simulink model "TST_PTOSwt_DD"  (R2016b)
settings: Solver=FixedStepDiscrete  StartTime=0.0  StopTime=0.1  FixedStep=sampleTime  RelTol=1e-3
values from neighbouring files (symbols this model uses):
  testCase = 1    [initTST_PTOSwt_DD_001.m]
libraries: simulink x2
settings Model: Creator=guofang02  LastModifiedBy=guofang02
settings DebuggingCC: SignalRangeChecking=error

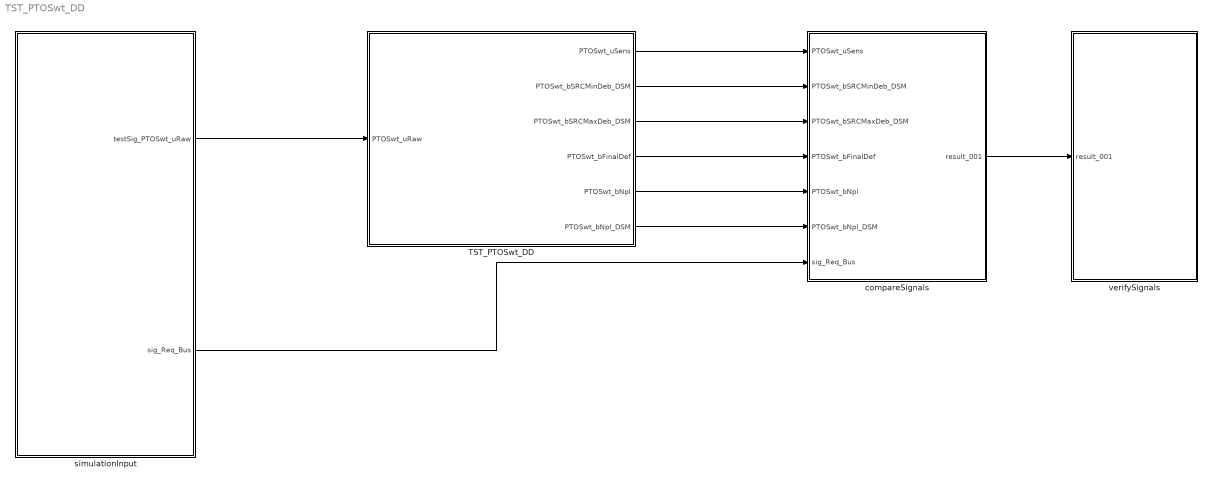
== system TST_PTOSwt_DD ==
  TST_PTOSwt_DD : Subsystem
  compareSignals : Subsystem
  simulationInput : Subsystem
  verifySignals : Subsystem
  wires:
  simulationInput/1(testSig_PTOSwt_uRaw) -> TST_PTOSwt_DD/1(PTOSwt_uRaw)
  TST_PTOSwt_DD/1(PTOSwt_uSens) -> compareSignals/1(PTOSwt_uSens)
  TST_PTOSwt_DD/2(PTOSwt_bSRCMinDeb_DSM) -> compareSignals/2(PTOSwt_bSRCMinDeb_DSM)
  TST_PTOSwt_DD/3(PTOSwt_bSRCMaxDeb_DSM) -> compareSignals/3(PTOSwt_bSRCMaxDeb_DSM)
  TST_PTOSwt_DD/4(PTOSwt_bFinalDef) -> compareSignals/4(PTOSwt_bFinalDef)
  TST_PTOSwt_DD/5(PTOSwt_bNpl) -> compareSignals/5(PTOSwt_bNpl)
  TST_PTOSwt_DD/6(PTOSwt_bNpl_DSM) -> compareSignals/6(PTOSwt_bNpl_DSM)
  simulationInput/2(sig_Req_Bus) -> compareSignals/7(sig_Req_Bus)
  compareSignals/1(result_001) -> verifySignals/1(result_001)

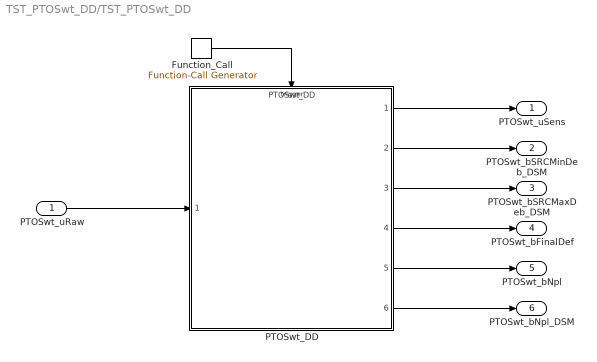
== system TST_PTOSwt_DD/TST_PTOSwt_DD ==
  PTOSwt_uRaw : Inport
  Function_Call : simulink/Ports & Subsystems/Function-Call Generator  sample_time=sampleTime  numberOfIterations=1
  PTOSwt_DD : ModelReference  ModelNameDialog=PTOSwt_DD  ModelReferenceVersion=1.16  TriggerPortName=function  TriggerPortTriggerType=function-call  TriggerPortStatesWhenEnabling=held
  PTOSwt_uSens : Outport
  PTOSwt_bSRCMinDeb_DSM : Outport  Port=2
  PTOSwt_bSRCMaxDeb_DSM : Outport  Port=3
  PTOSwt_bFinalDef : Outport  Port=4
  PTOSwt_bNpl : Outport  Port=5
  PTOSwt_bNpl_DSM : Outport  Port=6
  wires:
  Function_Call/1 -> PTOSwt_DD/Trigger
  PTOSwt_uRaw/1 -> PTOSwt_DD/1
  PTOSwt_DD/1 -> PTOSwt_uSens/1
  PTOSwt_DD/2 -> PTOSwt_bSRCMinDeb_DSM/1
  PTOSwt_DD/3 -> PTOSwt_bSRCMaxDeb_DSM/1
  PTOSwt_DD/4 -> PTOSwt_bFinalDef/1
  PTOSwt_DD/5 -> PTOSwt_bNpl/1
  PTOSwt_DD/6 -> PTOSwt_bNpl_DSM/1

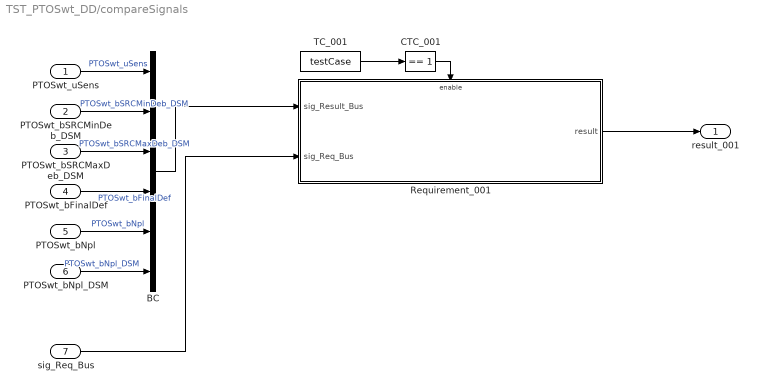
== system TST_PTOSwt_DD/compareSignals ==
  PTOSwt_uSens : Inport
  PTOSwt_bSRCMinDeb_DSM : Inport  Port=2
  PTOSwt_bSRCMaxDeb_DSM : Inport  Port=3
  PTOSwt_bFinalDef : Inport  Port=4
  PTOSwt_bNpl : Inport  Port=5
  PTOSwt_bNpl_DSM : Inport  Port=6
  sig_Req_Bus : Inport  Port=7
  BC : BusCreator  Inputs=6
  CTC_001 : simulink/Logic and Bit Operations/Compare To Constant  relop===  const=1  OutDataTypeStr=boolean
  Requirement_001 : Subsystem
  TC_001 : Constant  Value=testCase
  result_001 : Outport
  wires:
  PTOSwt_uSens/1 -> BC/1  "PTOSwt_uSens"
  PTOSwt_bSRCMinDeb_DSM/1 -> BC/2  "PTOSwt_bSRCMinDeb_DSM"
  PTOSwt_bSRCMaxDeb_DSM/1 -> BC/3  "PTOSwt_bSRCMaxDeb_DSM"
  PTOSwt_bFinalDef/1 -> BC/4  "PTOSwt_bFinalDef"
  PTOSwt_bNpl/1 -> BC/5  "PTOSwt_bNpl"
  PTOSwt_bNpl_DSM/1 -> BC/6  "PTOSwt_bNpl_DSM"
  TC_001/1 -> CTC_001/1
  CTC_001/1 -> Requirement_001/Enable
  sig_Req_Bus/1 -> Requirement_001/2(sig_Req_Bus)
  BC/1 -> Requirement_001/1(sig_Result_Bus)
  Requirement_001/1(result) -> result_001/1

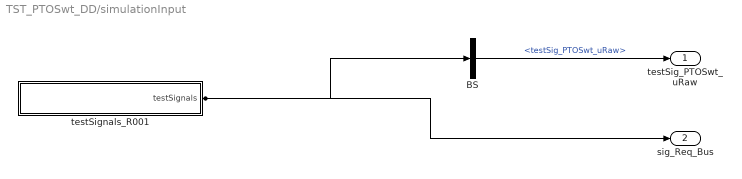
== system TST_PTOSwt_DD/simulationInput ==
  BS : BusSelector  OutputSignals=testSig_PTOSwt_uRaw
  testSignals_R001 : Subsystem
  testSig_PTOSwt_uRaw : Outport
  sig_Req_Bus : Outport  Port=2
  wires:
  BS/1 -> testSig_PTOSwt_uRaw/1  "<testSig_PTOSwt_uRaw>"
  testSignals_R001/1(testSignals) -> BS/1, sig_Req_Bus/1

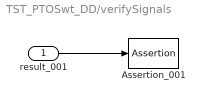
== system TST_PTOSwt_DD/verifySignals ==
  result_001 : Inport
  Assertion_001 : Assertion
  wires:
  result_001/1 -> Assertion_001/1

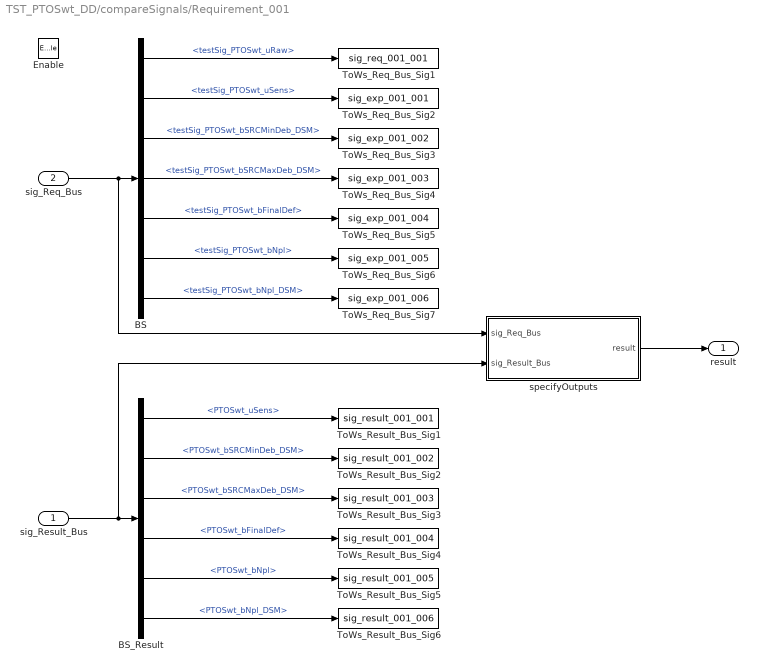
== system TST_PTOSwt_DD/compareSignals/Requirement_001 ==
  sig_Result_Bus : Inport
  sig_Req_Bus : Inport  Port=2
  Enable : EnablePort
  BS : BusSelector  OutputSignals=testSig_PTOSwt_uRaw,testSig_PTOSwt_uSens,testSig_PTOSwt_bSRCMinDeb_DSM,testSig_PTOSwt_bSRCMaxDeb_DSM,testSig_PTOSwt_bFinalDef,testSig_PTOSwt_bNpl,testSig_PTOSwt_bNpl_DSM
  BS_Result : BusSelector  OutputSignals=PTOSwt_uSens,PTOSwt_bSRCMinDeb_DSM,PTOSwt_bSRCMaxDeb_DSM,PTOSwt_bFinalDef,PTOSwt_bNpl,PTOSwt_bNpl_DSM
  ToWs_Req_Bus_Sig1 : ToWorkspace  VariableName=sig_req_001_001  SaveFormat=Structure With Time
  ToWs_Req_Bus_Sig2 : ToWorkspace  VariableName=sig_exp_001_001  SaveFormat=Structure With Time
  ToWs_Req_Bus_Sig3 : ToWorkspace  VariableName=sig_exp_001_002  SaveFormat=Structure With Time
  ToWs_Req_Bus_Sig4 : ToWorkspace  VariableName=sig_exp_001_003  SaveFormat=Structure With Time
  ToWs_Req_Bus_Sig5 : ToWorkspace  VariableName=sig_exp_001_004  SaveFormat=Structure With Time
  ToWs_Req_Bus_Sig6 : ToWorkspace  VariableName=sig_exp_001_005  SaveFormat=Structure With Time
  ToWs_Req_Bus_Sig7 : ToWorkspace  VariableName=sig_exp_001_006  SaveFormat=Structure With Time
  ToWs_Result_Bus_Sig1 : ToWorkspace  VariableName=sig_result_001_001  SaveFormat=Structure With Time
  ToWs_Result_Bus_Sig2 : ToWorkspace  VariableName=sig_result_001_002  SaveFormat=Structure With Time
  ToWs_Result_Bus_Sig3 : ToWorkspace  VariableName=sig_result_001_003  SaveFormat=Structure With Time
  ToWs_Result_Bus_Sig4 : ToWorkspace  VariableName=sig_result_001_004  SaveFormat=Structure With Time
  ToWs_Result_Bus_Sig5 : ToWorkspace  VariableName=sig_result_001_005  SaveFormat=Structure With Time
  ToWs_Result_Bus_Sig6 : ToWorkspace  VariableName=sig_result_001_006  SaveFormat=Structure With Time
  specifyOutputs : Subsystem
  result : Outport
  wires:
  sig_Req_Bus/1 -> BS/1, specifyOutputs/1(sig_Req_Bus)
  BS/1 -> ToWs_Req_Bus_Sig1/1  "<testSig_PTOSwt_uRaw>"
  BS/2 -> ToWs_Req_Bus_Sig2/1  "<testSig_PTOSwt_uSens>"
  BS/3 -> ToWs_Req_Bus_Sig3/1  "<testSig_PTOSwt_bSRCMinDeb_DSM>"
  BS/4 -> ToWs_Req_Bus_Sig4/1  "<testSig_PTOSwt_bSRCMaxDeb_DSM>"
  BS/5 -> ToWs_Req_Bus_Sig5/1  "<testSig_PTOSwt_bFinalDef>"
  BS/6 -> ToWs_Req_Bus_Sig6/1  "<testSig_PTOSwt_bNpl>"
  BS/7 -> ToWs_Req_Bus_Sig7/1  "<testSig_PTOSwt_bNpl_DSM>"
  sig_Result_Bus/1 -> BS_Result/1, specifyOutputs/2(sig_Result_Bus)
  BS_Result/1 -> ToWs_Result_Bus_Sig1/1  "<PTOSwt_uSens>"
  BS_Result/2 -> ToWs_Result_Bus_Sig2/1  "<PTOSwt_bSRCMinDeb_DSM>"
  BS_Result/3 -> ToWs_Result_Bus_Sig3/1  "<PTOSwt_bSRCMaxDeb_DSM>"
  BS_Result/4 -> ToWs_Result_Bus_Sig4/1  "<PTOSwt_bFinalDef>"
  BS_Result/5 -> ToWs_Result_Bus_Sig5/1  "<PTOSwt_bNpl>"
  BS_Result/6 -> ToWs_Result_Bus_Sig6/1  "<PTOSwt_bNpl_DSM>"
  specifyOutputs/1(result) -> result/1

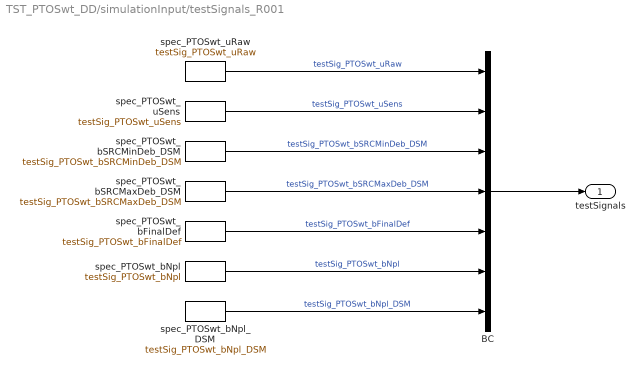
== system TST_PTOSwt_DD/simulationInput/testSignals_R001 ==
  BC : BusCreator  Inputs=7
  spec_PTOSwt_bFinalDef : FromWorkspace  VariableName=testSig_PTOSwt_bFinalDef  Interpolate=off  OutputAfterFinalValue=Holding final value
  spec_PTOSwt_bNpl : FromWorkspace  VariableName=testSig_PTOSwt_bNpl  Interpolate=off  OutputAfterFinalValue=Holding final value
  spec_PTOSwt_bNpl_DSM : FromWorkspace  VariableName=testSig_PTOSwt_bNpl_DSM  Interpolate=off  OutputAfterFinalValue=Holding final value
  spec_PTOSwt_bSRCMaxDeb_DSM : FromWorkspace  VariableName=testSig_PTOSwt_bSRCMaxDeb_DSM  Interpolate=off  OutputAfterFinalValue=Holding final value
  spec_PTOSwt_bSRCMinDeb_DSM : FromWorkspace  VariableName=testSig_PTOSwt_bSRCMinDeb_DSM  Interpolate=off  OutputAfterFinalValue=Holding final value
  spec_PTOSwt_uRaw : FromWorkspace  VariableName=testSig_PTOSwt_uRaw  Interpolate=off  OutputAfterFinalValue=Holding final value
  spec_PTOSwt_uSens : FromWorkspace  VariableName=testSig_PTOSwt_uSens  Interpolate=off  OutputAfterFinalValue=Holding final value
  testSignals : Outport
  wires:
  BC/1 -> testSignals/1
  spec_PTOSwt_uRaw/1 -> BC/1  "testSig_PTOSwt_uRaw"
  spec_PTOSwt_uSens/1 -> BC/2  "testSig_PTOSwt_uSens"
  spec_PTOSwt_bSRCMinDeb_DSM/1 -> BC/3  "testSig_PTOSwt_bSRCMinDeb_DSM"
  spec_PTOSwt_bSRCMaxDeb_DSM/1 -> BC/4  "testSig_PTOSwt_bSRCMaxDeb_DSM"
  spec_PTOSwt_bFinalDef/1 -> BC/5  "testSig_PTOSwt_bFinalDef"
  spec_PTOSwt_bNpl/1 -> BC/6  "testSig_PTOSwt_bNpl"
  spec_PTOSwt_bNpl_DSM/1 -> BC/7  "testSig_PTOSwt_bNpl_DSM"

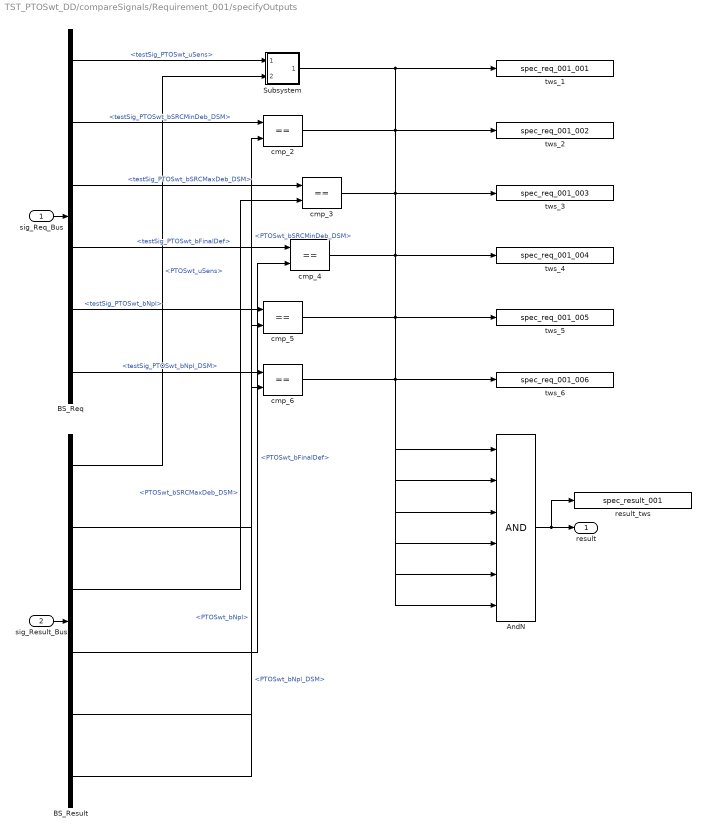
== system TST_PTOSwt_DD/compareSignals/Requirement_001/specifyOutputs ==
  sig_Req_Bus : Inport
  sig_Result_Bus : Inport  Port=2
  AndN : Logic  Inputs=6
  BS_Req : BusSelector  OutputSignals=testSig_PTOSwt_uSens,testSig_PTOSwt_bSRCMinDeb_DSM,testSig_PTOSwt_bSRCMaxDeb_DSM,testSig_PTOSwt_bFinalDef,testSig_PTOSwt_bNpl,testSig_PTOSwt_bNpl_DSM
  BS_Result : BusSelector  OutputSignals=PTOSwt_uSens,PTOSwt_bSRCMinDeb_DSM,PTOSwt_bSRCMaxDeb_DSM,PTOSwt_bFinalDef,PTOSwt_bNpl,PTOSwt_bNpl_DSM
  Subsystem : Subsystem
  cmp_{2..6} (5 alike) : RelationalOperator  Operator===  RndMeth=Nearest  InputSameDT=on
  result_tws : ToWorkspace  VariableName=spec_result_001
  tws_1 : ToWorkspace  VariableName=spec_req_001_001
  tws_2 : ToWorkspace  VariableName=spec_req_001_002
  tws_3 : ToWorkspace  VariableName=spec_req_001_003
  tws_4 : ToWorkspace  VariableName=spec_req_001_004
  tws_5 : ToWorkspace  VariableName=spec_req_001_005
  tws_6 : ToWorkspace  VariableName=spec_req_001_006
  result : Outport
  wires:
  sig_Req_Bus/1 -> BS_Req/1
  sig_Result_Bus/1 -> BS_Result/1
  AndN/1 -> result/1, result_tws/1
  BS_Req/1 -> Subsystem/1(In1)  "<testSig_PTOSwt_uSens>"
  BS_Result/1 -> Subsystem/2(In2)  "<PTOSwt_uSens>"
  Subsystem/1(Out1) -> tws_1/1, AndN/1
  BS_Req/2 -> cmp_2/1  "<testSig_PTOSwt_bSRCMinDeb_DSM>"
  BS_Result/2 -> cmp_2/2  "<PTOSwt_bSRCMinDeb_DSM>"
  cmp_2/1 -> tws_2/1, AndN/2
  BS_Req/3 -> cmp_3/1  "<testSig_PTOSwt_bSRCMaxDeb_DSM>"
  BS_Result/3 -> cmp_3/2  "<PTOSwt_bSRCMaxDeb_DSM>"
  cmp_3/1 -> tws_3/1, AndN/3
  BS_Req/4 -> cmp_4/1  "<testSig_PTOSwt_bFinalDef>"
  BS_Result/4 -> cmp_4/2  "<PTOSwt_bFinalDef>"
  cmp_4/1 -> tws_4/1, AndN/4
  BS_Req/5 -> cmp_5/1  "<testSig_PTOSwt_bNpl>"
  BS_Result/5 -> cmp_5/2  "<PTOSwt_bNpl>"
  cmp_5/1 -> tws_5/1, AndN/5
  BS_Req/6 -> cmp_6/1  "<testSig_PTOSwt_bNpl_DSM>"
  BS_Result/6 -> cmp_6/2  "<PTOSwt_bNpl_DSM>"
  cmp_6/1 -> tws_6/1, AndN/6

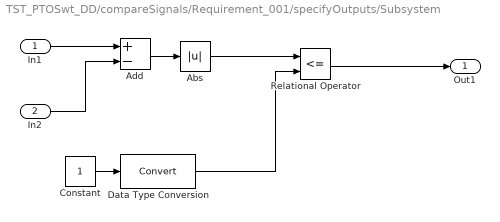
== system TST_PTOSwt_DD/compareSignals/Requirement_001/specifyOutputs/Subsystem ==
  In1 : Inport
  In2 : Inport  Port=2
  Abs : Abs
  Add : Sum  Inputs=+-
  Constant : Constant
  Data Type Conversion : DataTypeConversion
  Relational Operator : RelationalOperator  Operator=<=  OutDataTypeStr=boolean  RndMeth=Simplest
  Out1 : Outport
  wires:
  In1/1 -> Add/1
  In2/1 -> Add/2
  Constant/1 -> Data Type Conversion/1
  Add/1 -> Abs/1
  Data Type Conversion/1 -> Relational Operator/2
  Relational Operator/1 -> Out1/1
  Abs/1 -> Relational Operator/1
